simulink model "four_bit_subtractor"  (R2021a)
settings: Solver=VariableStepAuto  StartTime=0.0  StopTime=10.0  RelTol=1e-3
settings Model: Creator=kbhar  LastModifiedBy=kbhar

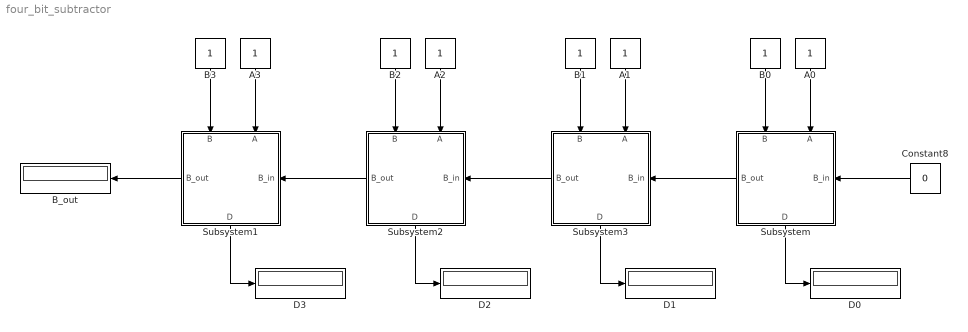
== system four_bit_subtractor ==
  A{0..3} (4 alike) : Constant
  B{0..3} (4 alike) : Constant
  B_out : Display
  Constant8 : Constant  Value=0
  D{0..3} (4 alike) : Display
  Subsystem : Subsystem
      settings: PortSchema="{\"entries\":[{\"content\":{\"sides\":[{\"content\":{\"connectorIds\":[\"In1\",\"In2\"]},\"type\":\"ConnectorPlacement.EquallySpacedRectSide\",\"uuid\":\"38d1d783-1e84-469f-b88f-34400794f458\"},{\"content\":{\"connectorIds\":[\"Out1\"],\"side\":\"RIGHT\"},\"type\":\"ConnectorPlacement.EquallySpacedRectSide\",\"uuid\":\"9549b396-3b16-432f-9c12-dae7a5b8dc11\"},{\"content\":{\"connectorIds\":[\"Out2\"],\"side\":\"TOP\"},\"type\":\"ConnectorPlacement.EquallySpacedRectSide\",\"uuid\":\"526a5790-86b3-4626-b4aa-b9520108ec40\"},{\"content\":{\"connectorIds\":[\"In3\"],\"side\":\"BOTTOM\"},\"type\":\"ConnectorPlacement.EquallySpacedRectSide\",\"uuid\":\"7b9a1b6a-14be-425f-b6da-6563ee756159\"}]},\"type\":\"ConnectorPlacement.EquallySpacedConnector\",\"uuid\":\"b57ea0ad-738f-4734-9daa-a65058de1f48\"}],\"packageUris\":[\"http://schema.mathworks.com/mf0/Connector/R2020b\"],\"version\":\"1.0\"}"
  Subsystem1 : Subsystem
      settings: PortSchema="{\"entries\":[{\"content\":{\"sides\":[{\"content\":{\"connectorIds\":[\"In1\",\"In2\"]},\"type\":\"ConnectorPlacement.EquallySpacedRectSide\",\"uuid\":\"38d1d783-1e84-469f-b88f-34400794f458\"},{\"content\":{\"connectorIds\":[\"Out1\"],\"side\":\"RIGHT\"},\"type\":\"ConnectorPlacement.EquallySpacedRectSide\",\"uuid\":\"9549b396-3b16-432f-9c12-dae7a5b8dc11\"},{\"content\":{\"connectorIds\":[\"Out2\"],\"side\":\"TOP\"},\"type\":\"ConnectorPlacement.EquallySpacedRectSide\",\"uuid\":\"526a5790-86b3-4626-b4aa-b9520108ec40\"},{\"content\":{\"connectorIds\":[\"In3\"],\"side\":\"BOTTOM\"},\"type\":\"ConnectorPlacement.EquallySpacedRectSide\",\"uuid\":\"7b9a1b6a-14be-425f-b6da-6563ee756159\"}]},\"type\":\"ConnectorPlacement.EquallySpacedConnector\",\"uuid\":\"b57ea0ad-738f-4734-9daa-a65058de1f48\"}],\"packageUris\":[\"http://schema.mathworks.com/mf0/Connector/R2020b\"],\"version\":\"1.0\"}"
  Subsystem2 : Subsystem
      settings: PortSchema="{\"entries\":[{\"content\":{\"sides\":[{\"content\":{\"connectorIds\":[\"In1\",\"In2\"]},\"type\":\"ConnectorPlacement.EquallySpacedRectSide\",\"uuid\":\"38d1d783-1e84-469f-b88f-34400794f458\"},{\"content\":{\"connectorIds\":[\"Out1\"],\"side\":\"RIGHT\"},\"type\":\"ConnectorPlacement.EquallySpacedRectSide\",\"uuid\":\"9549b396-3b16-432f-9c12-dae7a5b8dc11\"},{\"content\":{\"connectorIds\":[\"Out2\"],\"side\":\"TOP\"},\"type\":\"ConnectorPlacement.EquallySpacedRectSide\",\"uuid\":\"526a5790-86b3-4626-b4aa-b9520108ec40\"},{\"content\":{\"connectorIds\":[\"In3\"],\"side\":\"BOTTOM\"},\"type\":\"ConnectorPlacement.EquallySpacedRectSide\",\"uuid\":\"7b9a1b6a-14be-425f-b6da-6563ee756159\"}]},\"type\":\"ConnectorPlacement.EquallySpacedConnector\",\"uuid\":\"b57ea0ad-738f-4734-9daa-a65058de1f48\"}],\"packageUris\":[\"http://schema.mathworks.com/mf0/Connector/R2020b\"],\"version\":\"1.0\"}"
  Subsystem3 : Subsystem
      settings: PortSchema="{\"entries\":[{\"content\":{\"sides\":[{\"content\":{\"connectorIds\":[\"In1\",\"In2\"]},\"type\":\"ConnectorPlacement.EquallySpacedRectSide\",\"uuid\":\"38d1d783-1e84-469f-b88f-34400794f458\"},{\"content\":{\"connectorIds\":[\"Out1\"],\"side\":\"RIGHT\"},\"type\":\"ConnectorPlacement.EquallySpacedRectSide\",\"uuid\":\"9549b396-3b16-432f-9c12-dae7a5b8dc11\"},{\"content\":{\"connectorIds\":[\"Out2\"],\"side\":\"TOP\"},\"type\":\"ConnectorPlacement.EquallySpacedRectSide\",\"uuid\":\"526a5790-86b3-4626-b4aa-b9520108ec40\"},{\"content\":{\"connectorIds\":[\"In3\"],\"side\":\"BOTTOM\"},\"type\":\"ConnectorPlacement.EquallySpacedRectSide\",\"uuid\":\"7b9a1b6a-14be-425f-b6da-6563ee756159\"}]},\"type\":\"ConnectorPlacement.EquallySpacedConnector\",\"uuid\":\"b57ea0ad-738f-4734-9daa-a65058de1f48\"}],\"packageUris\":[\"http://schema.mathworks.com/mf0/Connector/R2020b\"],\"version\":\"1.0\"}"
  wires:
  Subsystem/2(B_out) -> Subsystem3/3(B_in)
  Subsystem3/2(B_out) -> Subsystem2/3(B_in)
  Subsystem2/2(B_out) -> Subsystem1/3(B_in)
  Subsystem/1(D) -> D0/1
  Subsystem1/1(D) -> D3/1
  Subsystem2/1(D) -> D2/1
  Subsystem3/1(D) -> D1/1
  Subsystem1/2(B_out) -> B_out/1
  B0/1 -> Subsystem/1(B)
  A0/1 -> Subsystem/2(A)
  B1/1 -> Subsystem3/1(B)
  A1/1 -> Subsystem3/2(A)
  A3/1 -> Subsystem1/2(A)
  B2/1 -> Subsystem2/1(B)
  A2/1 -> Subsystem2/2(A)
  B3/1 -> Subsystem1/1(B)
  Constant8/1 -> Subsystem/3(B_in)

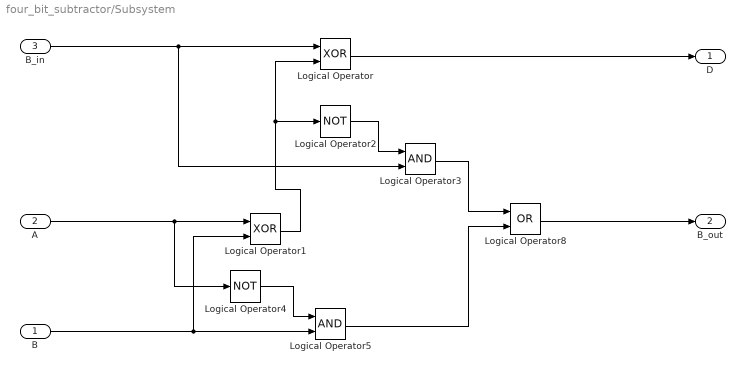
== system four_bit_subtractor/Subsystem ==
  B : Inport
  A : Inport  Port=2
  B_in : Inport  Port=3
  Logical Operator : Logic  Operator=XOR  AllPortsSameDT=off  OutDataTypeStr=boolean
  Logical Operator1 : Logic  Operator=XOR  AllPortsSameDT=off  OutDataTypeStr=boolean
  Logical Operator2 : Logic  Operator=NOT  AllPortsSameDT=off  OutDataTypeStr=boolean
  Logical Operator3 : Logic  AllPortsSameDT=off  OutDataTypeStr=boolean
  Logical Operator4 : Logic  Operator=NOT  AllPortsSameDT=off  OutDataTypeStr=boolean
  Logical Operator5 : Logic  AllPortsSameDT=off  OutDataTypeStr=boolean
  Logical Operator8 : Logic  Operator=OR  AllPortsSameDT=off  OutDataTypeStr=boolean
  D : Outport
  B_out : Outport  Port=2
  wires:
  Logical Operator2/1 -> Logical Operator3/1
  B_in/1 -> Logical Operator/1, Logical Operator3/2
  B/1 -> Logical Operator1/2, Logical Operator5/2
  Logical Operator1/1 -> Logical Operator2/1, Logical Operator/2
  A/1 -> Logical Operator1/1, Logical Operator4/1
  Logical Operator3/1 -> Logical Operator8/1
  Logical Operator5/1 -> Logical Operator8/2
  Logical Operator4/1 -> Logical Operator5/1
  Logical Operator/1 -> D/1
  Logical Operator8/1 -> B_out/1

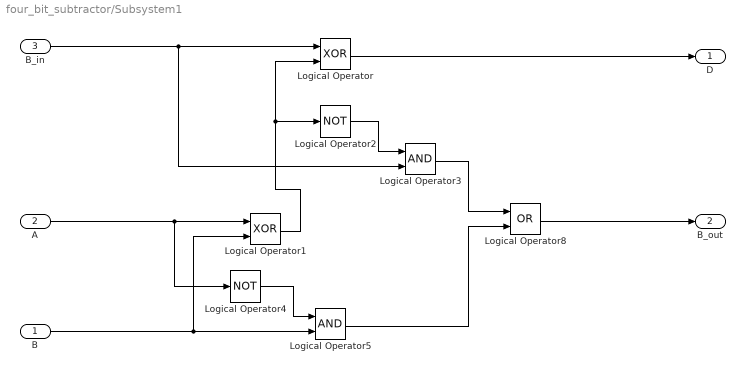
== system four_bit_subtractor/Subsystem1 ==
  B : Inport
  A : Inport  Port=2
  B_in : Inport  Port=3
  Logical Operator : Logic  Operator=XOR  AllPortsSameDT=off  OutDataTypeStr=boolean
  Logical Operator1 : Logic  Operator=XOR  AllPortsSameDT=off  OutDataTypeStr=boolean
  Logical Operator2 : Logic  Operator=NOT  AllPortsSameDT=off  OutDataTypeStr=boolean
  Logical Operator3 : Logic  AllPortsSameDT=off  OutDataTypeStr=boolean
  Logical Operator4 : Logic  Operator=NOT  AllPortsSameDT=off  OutDataTypeStr=boolean
  Logical Operator5 : Logic  AllPortsSameDT=off  OutDataTypeStr=boolean
  Logical Operator8 : Logic  Operator=OR  AllPortsSameDT=off  OutDataTypeStr=boolean
  D : Outport
  B_out : Outport  Port=2
  wires:
  Logical Operator2/1 -> Logical Operator3/1
  B_in/1 -> Logical Operator/1, Logical Operator3/2
  B/1 -> Logical Operator1/2, Logical Operator5/2
  Logical Operator1/1 -> Logical Operator2/1, Logical Operator/2
  A/1 -> Logical Operator1/1, Logical Operator4/1
  Logical Operator3/1 -> Logical Operator8/1
  Logical Operator5/1 -> Logical Operator8/2
  Logical Operator4/1 -> Logical Operator5/1
  Logical Operator/1 -> D/1
  Logical Operator8/1 -> B_out/1

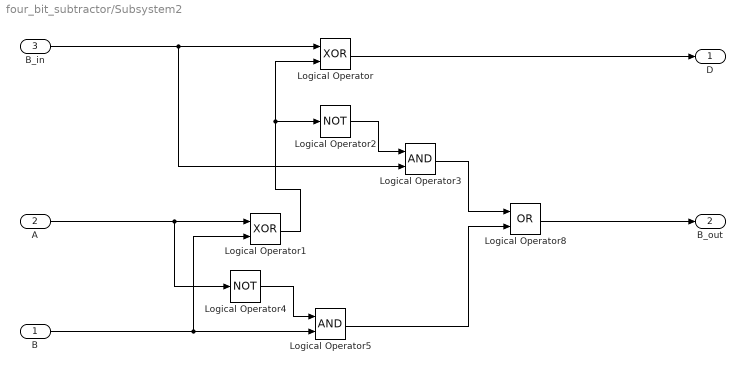
== system four_bit_subtractor/Subsystem2 ==
  B : Inport
  A : Inport  Port=2
  B_in : Inport  Port=3
  Logical Operator : Logic  Operator=XOR  AllPortsSameDT=off  OutDataTypeStr=boolean
  Logical Operator1 : Logic  Operator=XOR  AllPortsSameDT=off  OutDataTypeStr=boolean
  Logical Operator2 : Logic  Operator=NOT  AllPortsSameDT=off  OutDataTypeStr=boolean
  Logical Operator3 : Logic  AllPortsSameDT=off  OutDataTypeStr=boolean
  Logical Operator4 : Logic  Operator=NOT  AllPortsSameDT=off  OutDataTypeStr=boolean
  Logical Operator5 : Logic  AllPortsSameDT=off  OutDataTypeStr=boolean
  Logical Operator8 : Logic  Operator=OR  AllPortsSameDT=off  OutDataTypeStr=boolean
  D : Outport
  B_out : Outport  Port=2
  wires:
  Logical Operator2/1 -> Logical Operator3/1
  B_in/1 -> Logical Operator/1, Logical Operator3/2
  B/1 -> Logical Operator1/2, Logical Operator5/2
  Logical Operator1/1 -> Logical Operator2/1, Logical Operator/2
  A/1 -> Logical Operator1/1, Logical Operator4/1
  Logical Operator3/1 -> Logical Operator8/1
  Logical Operator5/1 -> Logical Operator8/2
  Logical Operator4/1 -> Logical Operator5/1
  Logical Operator/1 -> D/1
  Logical Operator8/1 -> B_out/1

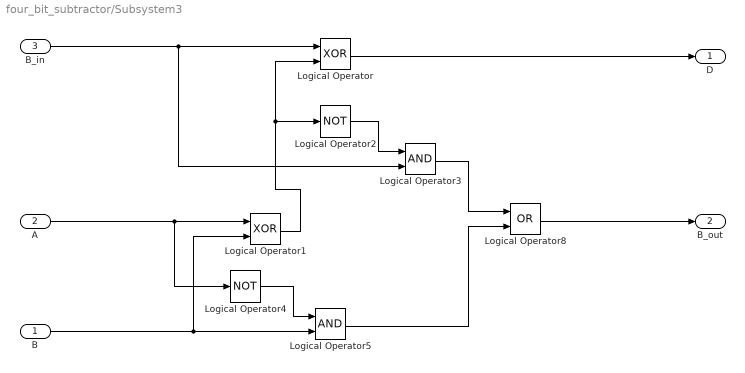
== system four_bit_subtractor/Subsystem3 ==
  B : Inport
  A : Inport  Port=2
  B_in : Inport  Port=3
  Logical Operator : Logic  Operator=XOR  AllPortsSameDT=off  OutDataTypeStr=boolean
  Logical Operator1 : Logic  Operator=XOR  AllPortsSameDT=off  OutDataTypeStr=boolean
  Logical Operator2 : Logic  Operator=NOT  AllPortsSameDT=off  OutDataTypeStr=boolean
  Logical Operator3 : Logic  AllPortsSameDT=off  OutDataTypeStr=boolean
  Logical Operator4 : Logic  Operator=NOT  AllPortsSameDT=off  OutDataTypeStr=boolean
  Logical Operator5 : Logic  AllPortsSameDT=off  OutDataTypeStr=boolean
  Logical Operator8 : Logic  Operator=OR  AllPortsSameDT=off  OutDataTypeStr=boolean
  D : Outport
  B_out : Outport  Port=2
  wires:
  Logical Operator2/1 -> Logical Operator3/1
  B_in/1 -> Logical Operator/1, Logical Operator3/2
  B/1 -> Logical Operator1/2, Logical Operator5/2
  Logical Operator1/1 -> Logical Operator2/1, Logical Operator/2
  A/1 -> Logical Operator1/1, Logical Operator4/1
  Logical Operator3/1 -> Logical Operator8/1
  Logical Operator5/1 -> Logical Operator8/2
  Logical Operator4/1 -> Logical Operator5/1
  Logical Operator/1 -> D/1
  Logical Operator8/1 -> B_out/1
